simulink model "CIGRE_Islanded_1SM_2GFM_1GFL"  (R2020b)
settings: Solver=FixedStepAuto  StartTime=0.0  StopTime=simlt.T_stop  RelTol=1e-3
undefined symbols (not defined in the file): simlt
libraries: G2ELib_V1 x55, powerlib x19, powerlib_meascontrol x13, eePowerMeasurement x13
(part 1 of 2)
settings Model: Creator=keladaf  LastModifiedBy=keladaf
settings DataIOCC: ReturnWorkspaceOutputs=off
settings DebuggingCC: UnconnectedInputMsg=none  UnconnectedOutputMsg=none  UnconnectedLineMsg=none

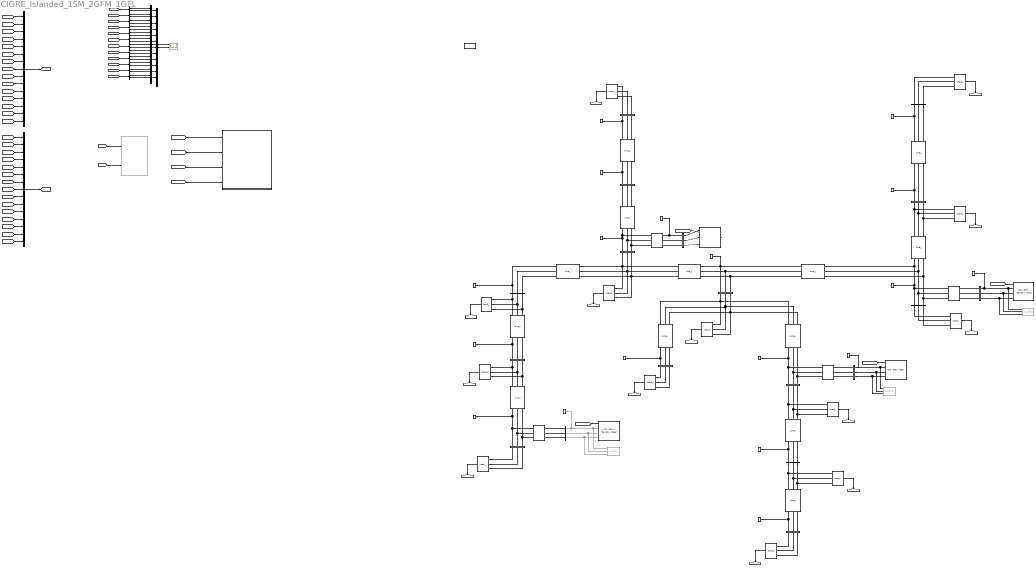
== system CIGRE_Islanded_1SM_2GFM_1GFL ==
  Bus Creator : BusCreator  Inputs=15
  Bus Creator1 : BusCreator  Inputs=15
  Bus Selector{,1..11} (12 alike) : BusSelector  OutputSignals=P_load,Q_load
  Bus_1 : G2ELib_V1/Miscellaneous Network Elements/Bus_i  VoltageMeasurement=phase-to-ground  SetLabelV=on  LabelV=V_Bus1  Vpu=off  VpuLL=off  CurrentMeasurement=yes  SetLabelI=on  LabelI=I_Bus1  Ipu=off  Pbase=100e6  Vbase=500e3  OutputType=Complex  PhasorSimulation=off  PSBequivalent=0
  Bus_10 : G2ELib_V1/Miscellaneous Network Elements/Bus_i  VoltageMeasurement=phase-to-ground  SetLabelV=on  LabelV=V_Bus10  Vpu=off  VpuLL=off  CurrentMeasurement=yes  SetLabelI=on  LabelI=I_Bus10  Ipu=off  Pbase=100e6  Vbase=500e3  OutputType=Complex  PhasorSimulation=off  PSBequivalent=0
  Bus_11 : G2ELib_V1/Miscellaneous Network Elements/Bus_i  VoltageMeasurement=phase-to-ground  SetLabelV=on  LabelV=V_Bus11  Vpu=off  VpuLL=off  CurrentMeasurement=yes  SetLabelI=on  LabelI=I_Bus11  Ipu=off  Pbase=100e6  Vbase=500e3  OutputType=Complex  PhasorSimulation=off  PSBequivalent=0
  Bus_12 : G2ELib_V1/Miscellaneous Network Elements/Bus_i  VoltageMeasurement=phase-to-ground  SetLabelV=on  LabelV=V_Bus12  Vpu=off  VpuLL=off  CurrentMeasurement=yes  SetLabelI=on  LabelI=I_Bus12  Ipu=off  Pbase=100e6  Vbase=500e3  OutputType=Complex  PhasorSimulation=off  PSBequivalent=0
  Bus_13 : G2ELib_V1/Miscellaneous Network Elements/Bus_i  VoltageMeasurement=phase-to-ground  SetLabelV=on  LabelV=V_Bus13  Vpu=off  VpuLL=off  CurrentMeasurement=yes  SetLabelI=on  LabelI=I_Bus13  Ipu=off  Pbase=100e6  Vbase=500e3  OutputType=Complex  PhasorSimulation=off  PSBequivalent=0
  Bus_14 : G2ELib_V1/Miscellaneous Network Elements/Bus_i  VoltageMeasurement=phase-to-ground  SetLabelV=on  LabelV=V_Bus14  Vpu=off  VpuLL=off  CurrentMeasurement=yes  SetLabelI=on  LabelI=I_Bus14  Ipu=off  Pbase=100e6  Vbase=500e3  OutputType=Complex  PhasorSimulation=off  PSBequivalent=0
  Bus_15 : G2ELib_V1/Miscellaneous Network Elements/Bus_i  VoltageMeasurement=phase-to-ground  SetLabelV=on  LabelV=V_Bus15  Vpu=off  VpuLL=off  CurrentMeasurement=yes  SetLabelI=on  LabelI=I_Bus15  Ipu=off  Pbase=100e6  Vbase=500e3  OutputType=Complex  PhasorSimulation=off  PSBequivalent=0
  Bus_16 : G2ELib_V1/Miscellaneous Network Elements/Bus_i  VoltageMeasurement=phase-to-ground  SetLabelV=on  LabelV=V_Bus16  Vpu=off  VpuLL=off  CurrentMeasurement=yes  SetLabelI=on  LabelI=I_Bus16  Ipu=off  Pbase=100e6  Vbase=500e3  OutputType=Complex  PhasorSimulation=off  PSBequivalent=0
  Bus_17 : G2ELib_V1/Miscellaneous Network Elements/Bus_i  VoltageMeasurement=phase-to-ground  SetLabelV=on  LabelV=V_Bus17  Vpu=off  VpuLL=off  CurrentMeasurement=yes  SetLabelI=on  LabelI=I_Bus17  Ipu=off  Pbase=100e6  Vbase=500e3  OutputType=Complex  PhasorSimulation=off  PSBequivalent=0
  Bus_18 : G2ELib_V1/Miscellaneous Network Elements/Bus_i  VoltageMeasurement=phase-to-ground  SetLabelV=on  LabelV=V_Bus18  Vpu=off  VpuLL=off  CurrentMeasurement=yes  SetLabelI=on  LabelI=I_Bus18  Ipu=off  Pbase=100e6  Vbase=500e3  OutputType=Complex  PhasorSimulation=off  PSBequivalent=0
  Bus_2 : G2ELib_V1/Miscellaneous Network Elements/Bus_i  VoltageMeasurement=phase-to-ground  SetLabelV=on  LabelV=V_Bus2  Vpu=off  VpuLL=off  CurrentMeasurement=yes  SetLabelI=on  LabelI=I_Bus2  Ipu=off  Pbase=100e6  Vbase=500e3  OutputType=Complex  PhasorSimulation=off  PSBequivalent=0
  Bus_3 : G2ELib_V1/Miscellaneous Network Elements/Bus_i  VoltageMeasurement=phase-to-ground  SetLabelV=on  LabelV=V_Bus3  Vpu=off  VpuLL=off  CurrentMeasurement=yes  SetLabelI=on  LabelI=I_Bus3  Ipu=off  Pbase=100e6  Vbase=500e3  OutputType=Complex  PhasorSimulation=off  PSBequivalent=0
  Bus_4 : G2ELib_V1/Miscellaneous Network Elements/Bus_i  VoltageMeasurement=phase-to-ground  SetLabelV=on  LabelV=V_Bus4  Vpu=off  VpuLL=off  CurrentMeasurement=yes  SetLabelI=on  LabelI=I_Bus4  Ipu=off  Pbase=100e6  Vbase=500e3  OutputType=Complex  PhasorSimulation=off  PSBequivalent=0
  Bus_5 : G2ELib_V1/Miscellaneous Network Elements/Bus_i  VoltageMeasurement=phase-to-ground  SetLabelV=on  LabelV=V_Bus5  Vpu=off  VpuLL=off  CurrentMeasurement=yes  SetLabelI=on  LabelI=I_Bus5  Ipu=off  Pbase=100e6  Vbase=500e3  OutputType=Complex  PhasorSimulation=off  PSBequivalent=0
  Bus_6 : G2ELib_V1/Miscellaneous Network Elements/Bus_i  VoltageMeasurement=phase-to-ground  SetLabelV=on  LabelV=V_Bus6  Vpu=off  VpuLL=off  CurrentMeasurement=yes  SetLabelI=on  LabelI=I_Bus6  Ipu=off  Pbase=100e6  Vbase=500e3  OutputType=Complex  PhasorSimulation=off  PSBequivalent=0
  Bus_7 : G2ELib_V1/Miscellaneous Network Elements/Bus_i  VoltageMeasurement=phase-to-ground  SetLabelV=on  LabelV=V_Bus7  Vpu=off  VpuLL=off  CurrentMeasurement=yes  SetLabelI=on  LabelI=I_Bus7  Ipu=off  Pbase=100e6  Vbase=500e3  OutputType=Complex  PhasorSimulation=off  PSBequivalent=0
  Bus_8 : G2ELib_V1/Miscellaneous Network Elements/Bus_i  VoltageMeasurement=phase-to-ground  SetLabelV=on  LabelV=V_Bus8  Vpu=off  VpuLL=off  CurrentMeasurement=yes  SetLabelI=on  LabelI=I_Bus8  Ipu=off  Pbase=100e6  Vbase=500e3  OutputType=Complex  PhasorSimulation=off  PSBequivalent=0
  Bus_9 : G2ELib_V1/Miscellaneous Network Elements/Bus_i  VoltageMeasurement=phase-to-ground  SetLabelV=on  LabelV=V_Bus9  Vpu=off  VpuLL=off  CurrentMeasurement=yes  SetLabelI=on  LabelI=I_Bus9  Ipu=off  Pbase=100e6  Vbase=500e3  OutputType=Complex  PhasorSimulation=off  PSBequivalent=0
  GFL_1 : G2ELib_V1/DC//AC Converters/Voltage Source Converters (VSC)/Grid-Following VSC (GFL)/VSC - GFL - Ideal  index_c=1  Parameters_fb=50  Parameters_wb=314.1593  GFL_Un=10000  GFL_Un_dc=16329.9316  GFL_Sn=2500000  GFL_Ib=204.1241  GFL_Ub=8164.9658  GFL_Ub_dc=16329.9316  GFL_Ib_dc=153.0931  GFL_Pref=0.7  GFL_Qref=0  GFL_V=0.98868  GFL_Theta_Eg0=-0.0027438  GFL_Vdcref=16329.9316  Delta_Pref_GFL=0.1  Tsw_Pref_GFL=1  Delta_Qref_GFL=0.1  Tsw_Qref_GFL=200  GFL_DC_link_R=500000  GFL_DC_link_C=0.05  GFL_DC_link_Vdc_init=16329.9316  DC_link_Tdc=1e-3  GFL_R1_pu=0.015  GFL_R2_pu=0.0533  GFL_L1_pu=0.1  GFL_L2_pu=0.00061115  GFL_C_pu=0.11  GFL_R1=0.6  GFL_R2=2.132  GFL_L1=0.012732  GFL_L2=7.7814e-05  GFL_C=8.7535e-06  Controllers=PLL  GFL_Control_PLL=1  GFL_Control_VIM=0  GFL_Control_SU_theta=1  GFL_Control_SU_omega=1  GFL_vdc_Kp=-319.9998  GFL_vdc_Ki=-9602.9001  GFL_KQ=-30  GFL_Inner_current_loop_Kp=0.17599  GFL_Inner_current_loop_Ki=57.3131  GFL_Inner_current_loop_Kffv=1  PLL_Kp=0.38197  PLL_Ki=22.9252  M_pll_0=-0.04362  VIM_wc=15.708  VIM_wc_ini=0  VIM_Iqd_sat=0.25  VIM_Rr_pu=0.0005  VIM_Lr_pu=0.05  VIM_Lm_pu=0.6  VIM_Rr=0.02  VIM_Lr=0.0063662  VIM_Lm=0.076394  VIM_Kp=3.1416  VIM_Kd=0.001  VIM_Nd=100  VIM_H=5.04  VIM_J=0.00025533  VIM_D=0.8  VIM_Inertia_ini=0  VIM_Ke_ini=0  VIM_T_sync=0  VIM_f0=50  VIM_w0=1  GFL_Inner_current_loop_Int_ini_d=0.01062  GFL_Inner_current_loop_Int_ini_q=0.0016313  GFL_Filter_I_ini="[ 21.80285     -136.1143      114.3114 ]"  GFL_Filter_V_ini="[ -22.149109     -6979.9183      7002.0674 ]"  GFL_Line_I_ini="[ -0.3965366     -124.9618      125.3584 ]"  GFL_Is0_dq0="[ 0.70802     0.10875           0 ]"  GFL_Eg0_dq0="[ 0.98868           0           0 ]"  GFL_Ig0_dq0="[ 0.70802           0           0 ]"  GFL_Vm0_dq0="[ 0.98842    0.072433           0 ]"  M_d_0=-7.3729e-05  M_q_0=-0.0036252  GFL_theta=-0.0027438
  GFM_1 : G2ELib_V1/DC//AC Converters/Voltage Source Converters (VSC)/Grid-Forming VSC (GFM)/VSC - GFM - Generic - Ideal  index_c=1  Parameters_fb=50  Parameters_wb=314.1593  GFM_Un=10000  GFM_Un_dc=16329.9316  GFM_Sn=2500000  GFM_Ib=204.1241  GFM_Ub=8164.9658  GFM_Ub_dc=16329.9316  GFM_Ib_dc=153.0931  GFM_Pref=0.7  GFM_Qref=0.40224  GFM_Vref=1  GFM_Theta_Eg0=-0.0039351  GFM_Vdcref=16329.9316  Delta_Pref_GFM=-0.1  Tsw_Pref_GFM=2  Delta_Vref_GFM=-0.01  Tsw_Vref_GFM=300  DC_link_R=500000  DC_link_C=0.05  DC_link_Vdc_init=16329.9316  DC_link_Tdc=1e-3  GFM_R1_pu=0.01  GFM_R2_pu=0.0533  GFM_L1_pu=0.1  GFM_L2_pu=0.00061115  GFM_C_pu=0.1  GFM_R1=0.4  GFM_R2=2.132  GFM_L1=0.012732  GFM_L2=7.7814e-05  GFM_C=7.9577e-06  Controllers=Droop  Control_PLL=0  Control_VIM=0  Control_MMU_QVDroop=1  Control_MMU_VSM=0  Control_dVOC=0  Control_MMU=1  Control_SU_PfDroop=1  Control_SU_Matching=0  Control_SU_VSM=0  Control_SU_theta=2  Control_SU_omega=2  Control_omega_set=2  Droop_mp=0.035  Droop_nq=0.0001  Droop_wc=2.5762  Droop_Int_ini=0  q_filter_wf=31.4159  q_filter_Int_ini=0.40224  p_filter_Int_ini=0.7  dVOC_eta=0.035  dVOC_alpha=5000  Matching_K_theta=112  VSM_D=28.5714  VSM_J=0.90946  VSM_AVR_Kp=0.05  VSM_AVR_Ki=11.64  VSM_Dq=10000  VSM_K=318.3099  Vdc_loop_Ki=0  Vdc_loop_Kp=3199.9998  Vdc_loop_Kffi=1  Vdc_loop_Int_ini=16329.9316  Damping_resistor_Enable=0  Damping_resistor_Rv=-0.052947  Damping_resistor_W_RV=62.8319  VI_Enable=0  VI_Rv_pu=0.01  VI_Lv_pu=0.1  TVI_K_RV=0.60041  TVI_Rho_XR=5  TVI_I_thresh_pu=1.2  Inner_voltage_loop_Kp=0.12732  Inner_voltage_loop_Ki=25.4725  Inner_voltage_loop_Kffi=1  Inner_current_loop_Kp=19.0886  Inner_current_loop_Ki=573130.8807  Inner_current_loop_Kffv=1  PLL_Kp=0.4  PLL_Ki=4.69  PLL_Int_ini=0  VIM_wc=0.1*2*pi*50  VIM_wc_ini=0  VIM_Iqd_sat=0.25  VIM_Rr_pu=0.0005  VIM_Lr_pu=0.05  VIM_Lm_pu=0.6  VIM_Rr=0.0048  VIM_Lr=0.0015  VIM_Lm=0.0183  VIM_Kp=3.1416  VIM_Kd=0.001  VIM_Nd=100  VIM_H=0  VIM_J=0.0043  VIM_D=10  VIM_Inertia_ini=0  VIM_Ke_ini=0  VIM_T_sync=0.01  VIM_f0=50.08  VIM_w0=1.0016  SFR_Enable=0  SFR_Rc=0.001  SFR_dP_max=0.3  Inner_voltage_loop_Int_ini_d=0  Inner_voltage_loop_Int_ini_q=-1.3878e-17  Inner_current_loop_Int_ini_d=0.007  Inner_current_loop_Int_ini_q=-0.0030224  Damping_resistor_Int_ini=0  Filter_I_ini="[ -62.25724     -92.40386      154.6611 ]"  Filter_V_ini="[ -32.129855     -7054.9481       7087.078 ]"  Line_I_ini="[ -82.6695     -82.12817      164.7977 ]"  Is0_dq0="[ 0.7    -0.30224           0 ]"  Eg0_dq0="[ 1           0           0 ]"  Ig0_dq0="[ 0.7    -0.40224           0 ]"  Vm0_dq0="[ 1.0372    0.066978           0 ]"  dVOC_ini_theta=-0.0039351  dVOC_ini_R0=[1,0;0,1]  Matching_Int_ini=-0.0039351  GFM_theta=-0.0039351
  GFM_2 : G2ELib_V1/DC//AC Converters/Voltage Source Converters (VSC)/Grid-Forming VSC (GFM)/VSC - GFM - Generic - Ideal  index_c=2  Parameters_fb=50  Parameters_wb=314.1593  GFM_Un=10000  GFM_Un_dc=16329.9316  GFM_Sn=2500000  GFM_Ib=204.1241  GFM_Ub=8164.9658  GFM_Ub_dc=16329.9316  GFM_Ib_dc=153.0931  GFM_Pref=0.7  GFM_Qref=0.20978  GFM_Vref=1  GFM_Theta_Eg0=0.0013498  GFM_Vdcref=16329.9316  Delta_Pref_GFM=-0.1  Tsw_Pref_GFM=2  Delta_Vref_GFM=-0.01  Tsw_Vref_GFM=300  DC_link_R=500000  DC_link_C=0.05  DC_link_Vdc_init=16329.9316  DC_link_Tdc=1e-3  GFM_R1_pu=0.01  GFM_R2_pu=0.0533  GFM_L1_pu=0.1  GFM_L2_pu=0.00061115  GFM_C_pu=0.1  GFM_R1=0.4  GFM_R2=2.132  GFM_L1=0.012732  GFM_L2=7.7814e-05  GFM_C=7.9577e-06  Controllers=Droop  Control_PLL=0  Control_VIM=0  Control_MMU_QVDroop=1  Control_MMU_VSM=0  Control_dVOC=0  Control_MMU=1  Control_SU_PfDroop=1  Control_SU_Matching=0  Control_SU_VSM=0  Control_SU_theta=2  Control_SU_omega=2  Control_omega_set=2  Droop_mp=0.035  Droop_nq=0.0001  Droop_wc=2.5762  Droop_Int_ini=0  q_filter_wf=31.4159  q_filter_Int_ini=0.20978  p_filter_Int_ini=0.7  dVOC_eta=0.035  dVOC_alpha=5000  Matching_K_theta=112  VSM_D=28.5714  VSM_J=0.90946  VSM_AVR_Kp=0.05  VSM_AVR_Ki=11.64  VSM_Dq=10000  VSM_K=318.3099  Vdc_loop_Ki=0  Vdc_loop_Kp=3199.9998  Vdc_loop_Kffi=1  Vdc_loop_Int_ini=16329.9316  Damping_resistor_Enable=0  Damping_resistor_Rv=-0.052947  Damping_resistor_W_RV=62.8319  VI_Enable=0  VI_Rv_pu=0.01  VI_Lv_pu=0.1  TVI_K_RV=0.60041  TVI_Rho_XR=5  TVI_I_thresh_pu=1.2  Inner_voltage_loop_Kp=0.12732  Inner_voltage_loop_Ki=25.4725  Inner_voltage_loop_Kffi=1  Inner_current_loop_Kp=19.0886  Inner_current_loop_Ki=573130.8807  Inner_current_loop_Kffv=1  PLL_Kp=0.4  PLL_Ki=4.69  PLL_Int_ini=0  VIM_wc=0.1*2*pi*50  VIM_wc_ini=0  VIM_Iqd_sat=0.25  VIM_Rr_pu=0.0005  VIM_Lr_pu=0.05  VIM_Lm_pu=0.6  VIM_Rr=0.0048  VIM_Lr=0.0015  VIM_Lm=0.0183  VIM_Kp=3.1416  VIM_Kd=0.001  VIM_Nd=100  VIM_H=0  VIM_J=0.0043  VIM_D=10  VIM_Inertia_ini=0  VIM_Ke_ini=0  VIM_T_sync=0.01  VIM_f0=50.08  VIM_w0=1.0016  SFR_Enable=0  SFR_Rc=0.001  SFR_dP_max=0.3  Inner_voltage_loop_Int_ini_d=0  Inner_voltage_loop_Int_ini_q=0  Inner_current_loop_Int_ini_d=0.007  Inner_current_loop_Int_ini_q=-0.0010978  Damping_resistor_Int_ini=0  Filter_I_ini="[ -22.21578     -112.6619      134.8777 ]"  Filter_V_ini="[ 11.021263      -7076.572      7065.5507 ]"  Line_I_ini="[ -42.62818     -102.4795      145.1077 ]"  Is0_dq0="[ 0.7    -0.10978           0 ]"  Eg0_dq0="[ 1  0  0 ]"  Ig0_dq0="[ 0.7    -0.20978           0 ]"  Vm0_dq0="[ 1.018    0.068902           0 ]"  dVOC_ini_theta=0.0013498  dVOC_ini_R0=[1,0;0,1]  Matching_Int_ini=0.0013498  GFM_theta=0.0013498
  Init_GFL_1 : G2ELib_V1/DC//AC Converters/Voltage Source Converters (VSC)/Grid-Following VSC (GFL)/Init_GFL_i  Commented=on  InternalConnection=Yg  VoltagePhases=off  Voltage=(10000)*0.988601  PhaseAngle=-0.17273  Voltage_phases=[25e3 25e3 25e3]/sqrt(3)  PhaseAngles_phases=[0 -120 +120]  Frequency=50  NonIdealSource=off  SpecifyImpedance=off  Resistance=0.8929  Inductance=16.58e-3  ShortCircuitLevel=100e6  BaseVoltage=10000  XRratio=7  BusType=PQ  Pref=1750000  Qref=0  Prefabc=[10e3, 10e3, 10e3]  Qrefabc=[0, 0, 0]  Qmin=-inf  Qmax=inf
  Init_GFM_1 : G2ELib_V1/DC//AC Converters/Voltage Source Converters (VSC)/Grid-Forming VSC (GFM)/Init_GFM_i  Commented=on  InternalConnection=Yg  VoltagePhases=off  Voltage=(10000)*1  PhaseAngle=-0.24228  Voltage_phases=[25e3 25e3 25e3]/sqrt(3)  PhaseAngles_phases=[0 -120 +120]  Frequency=50  NonIdealSource=off  SpecifyImpedance=off  Resistance=0.8929  Inductance=16.58e-3  ShortCircuitLevel=100e6  BaseVoltage=10000  XRratio=7  BusType=PV  Pref=1750000  Qref=1005611.7894  Prefabc=[10e3, 10e3, 10e3]  Qrefabc=[0, 0, 0]  Qmin=-inf  Qmax=inf
  Init_GFM_2 : G2ELib_V1/DC//AC Converters/Voltage Source Converters (VSC)/Grid-Forming VSC (GFM)/Init_GFM_i  Commented=on  InternalConnection=Yg  VoltagePhases=off  Voltage=(10000)*1  PhaseAngle=0.061558  Voltage_phases=[25e3 25e3 25e3]/sqrt(3)  PhaseAngles_phases=[0 -120 +120]  Frequency=50  NonIdealSource=off  SpecifyImpedance=off  Resistance=0.8929  Inductance=16.58e-3  ShortCircuitLevel=100e6  BaseVoltage=10000  XRratio=7  BusType=PV  Pref=1750000  Qref=524449.1246  Prefabc=[10e3, 10e3, 10e3]  Qrefabc=[0, 0, 0]  Qmin=-inf  Qmax=inf
  Line_1 : G2ELib_V1/Miscellaneous Network Elements/Line_i  LConnTagsString=a|b|c  RConnTagsString=A|B|C  Length=2.82  Frequency=50  Resistances=[ 0.501 0.3864 ]  Inductances=[ 0.0022791 0.0041264 ]  Capacitances=[ 1.5117e-07 7.751e-09 ]
      settings: AttributesFormatString=\n
  Line_10 : G2ELib_V1/Miscellaneous Network Elements/Line_i  LConnTagsString=a|b|c  RConnTagsString=A|B|C  Length=0.32  Frequency=50  Resistances=[ 0.501 0.3864 ]  Inductances=[ 0.0022791 0.0041264 ]  Capacitances=[ 1.5117e-07 7.751e-09 ]
      settings: AttributesFormatString=\n
  Line_11 : G2ELib_V1/Miscellaneous Network Elements/Line_i  LConnTagsString=a|b|c  RConnTagsString=A|B|C  Length=4.89  Frequency=50  Resistances=[ 0.51 0.3864 ]  Inductances=[ 0.001165 0.0041264 ]  Capacitances=[ 1.0097e-08 7.751e-09 ]
      settings: AttributesFormatString=\n
  Line_12 : G2ELib_V1/Miscellaneous Network Elements/Line_i  LConnTagsString=a|b|c  RConnTagsString=A|B|C  Length=2.99  Frequency=50  Resistances=[ 0.51 0.3864 ]  Inductances=[ 0.001165 0.0041264 ]  Capacitances=[ 1.0097e-08 7.751e-09 ]
      settings: AttributesFormatString=\n
  Line_13 : G2ELib_V1/Miscellaneous Network Elements/Line_i  LConnTagsString=a|b|c  RConnTagsString=A|B|C  Length=2  Frequency=50  Resistances=[ 0.51 0.3864 ]  Inductances=[ 0.001165 0.0041264 ]  Capacitances=[ 1.0097e-08 7.751e-09 ]
      settings: AttributesFormatString=\n
  Line_2 : G2ELib_V1/Miscellaneous Network Elements/Line_i  LConnTagsString=a|b|c  RConnTagsString=A|B|C  Length=4.42  Frequency=50  Resistances=[ 0.501 0.3864 ]  Inductances=[ 0.0022791 0.0041264 ]  Capacitances=[ 1.5117e-07 7.751e-09 ]
      settings: AttributesFormatString=\n
  Line_3 : G2ELib_V1/Miscellaneous Network Elements/Line_i  LConnTagsString=a|b|c  RConnTagsString=A|B|C  Length=0.61  Frequency=50  Resistances=[ 0.501 0.3864 ]  Inductances=[ 0.0022791 0.0041264 ]  Capacitances=[ 1.5117e-07 7.751e-09 ]
      settings: AttributesFormatString=\n
  Line_4 : G2ELib_V1/Miscellaneous Network Elements/Line_i  LConnTagsString=a|b|c  RConnTagsString=A|B|C  Length=0.56  Frequency=50  Resistances=[ 0.501 0.3864 ]  Inductances=[ 0.0022791 0.0041264 ]  Capacitances=[ 1.5117e-07 7.751e-09 ]
      settings: AttributesFormatString=\n
  Line_5 : G2ELib_V1/Miscellaneous Network Elements/Line_i  LConnTagsString=a|b|c  RConnTagsString=A|B|C  Length=1.54  Frequency=50  Resistances=[ 0.501 0.3864 ]  Inductances=[ 0.0022791 0.0041264 ]  Capacitances=[ 1.5117e-07 7.751e-09 ]
      settings: AttributesFormatString=\n
  Line_6 : G2ELib_V1/Miscellaneous Network Elements/Line_i  LConnTagsString=a|b|c  RConnTagsString=A|B|C  Length=1.3  Frequency=50  Resistances=[ 0.501 0.3864 ]  Inductances=[ 0.0022791 0.0041264 ]  Capacitances=[ 1.5117e-07 7.751e-09 ]
      settings: AttributesFormatString=\n
  Line_7 : G2ELib_V1/Miscellaneous Network Elements/Line_i  LConnTagsString=a|b|c  RConnTagsString=A|B|C  Length=1.67  Frequency=50  Resistances=[ 0.501 0.3864 ]  Inductances=[ 0.0022791 0.0041264 ]  Capacitances=[ 1.5117e-07 7.751e-09 ]
      settings: AttributesFormatString=\n
  Line_8 : G2ELib_V1/Miscellaneous Network Elements/Line_i  LConnTagsString=a|b|c  RConnTagsString=A|B|C  Length=0.24  Frequency=50  Resistances=[ 0.501 0.3864 ]  Inductances=[ 0.0022791 0.0041264 ]  Capacitances=[ 1.5117e-07 7.751e-09 ]
      settings: AttributesFormatString=\n
  Line_9 : G2ELib_V1/Miscellaneous Network Elements/Line_i  LConnTagsString=a|b|c  RConnTagsString=A|B|C  Length=0.77  Frequency=50  Resistances=[ 0.501 0.3864 ]  Inductances=[ 0.0022791 0.0041264 ]  Capacitances=[ 1.5117e-07 7.751e-09 ]
      settings: AttributesFormatString=\n
  Load Flow Bus1 : powerlib/Measurements/Load Flow Bus  LConnTagsString=a  Phases=single  Connectors=on one side  ID=BUS_1  Vbase=20000  Vref=1  Vangle=0  VLF=0.9759  VLFb=1  VLFc=1  angleLF=-1.897  angleLFb=0  angleLFc=0
  Load Flow Bus10 : powerlib/Measurements/Load Flow Bus  LConnTagsString=a  Phases=single  Connectors=on one side  ID=BUS_10  Vbase=20000  Vref=1  Vangle=0  VLF=0.9869  VLFb=1  VLFc=1  angleLF=-1.245  angleLFb=0  angleLFc=0
  Load Flow Bus11 : powerlib/Measurements/Load Flow Bus  LConnTagsString=a  Phases=single  Connectors=on one side  ID=BUS_11  Vbase=20000  Vref=1  Vangle=0  VLF=0.9865  VLFb=1  VLFc=1  angleLF=-1.266  angleLFb=0  angleLFc=0
  Load Flow Bus12 : powerlib/Measurements/Load Flow Bus  LConnTagsString=a  Phases=single  Connectors=on one side  ID=BUS_12  Vbase=20000  Vref=1  Vangle=0  VLF=0.9903  VLFb=1  VLFc=1  angleLF=-1.208  angleLFb=0  angleLFc=0
  Load Flow Bus13 : powerlib/Measurements/Load Flow Bus  LConnTagsString=a  Phases=single  Connectors=on one side  ID=BUS_13  Vbase=20000  Vref=1  Vangle=0  VLF=0.9839  VLFb=1  VLFc=1  angleLF=-1.348  angleLFb=0  angleLFc=0
  Load Flow Bus14 : powerlib/Measurements/Load Flow Bus  LConnTagsString=a  Phases=single  Connectors=on one side  ID=BUS_14  Vbase=20000  Vref=1  Vangle=0  VLF=0.9802  VLFb=1  VLFc=1  angleLF=-1.432  angleLFb=0  angleLFc=0
  Load Flow Bus15 : powerlib/Measurements/Load Flow Bus  LConnTagsString=a  Phases=single  Connectors=on one side  ID=BUS_15  Vbase=10000  Vref=1  Vangle=0  VLF=1  VLFb=1  VLFc=1  angleLF=0  angleLFb=0  angleLFc=0
  Load Flow Bus16 : powerlib/Measurements/Load Flow Bus  LConnTagsString=a  Phases=single  Connectors=on one side  ID=BUS_16  Vbase=10000  Vref=1  Vangle=0  VLF=1  VLFb=1  VLFc=1  angleLF=-0.2423  angleLFb=0  angleLFc=0
  Load Flow Bus17 : powerlib/Measurements/Load Flow Bus  LConnTagsString=a  Phases=single  Connectors=on one side  ID=BUS_17  Vbase=10000  Vref=1  Vangle=0  VLF=1  VLFb=1  VLFc=1  angleLF=0.06156  angleLFb=0  angleLFc=0
  Load Flow Bus18 : powerlib/Measurements/Load Flow Bus  LConnTagsString=a  Phases=single  Connectors=on one side  ID=BUS_18  Vbase=10000  Vref=1  Vangle=0  VLF=0.9886  VLFb=1  VLFc=1  angleLF=-0.1727  angleLFb=0  angleLFc=0
  Load Flow Bus2 : powerlib/Measurements/Load Flow Bus  LConnTagsString=a  Phases=single  Connectors=on one side  ID=BUS_2  Vbase=20000  Vref=1  Vangle=0  VLF=0.9819  VLFb=1  VLFc=1  angleLF=-1.603  angleLFb=0  angleLFc=0
  Load Flow Bus3 : powerlib/Measurements/Load Flow Bus  LConnTagsString=a  Phases=single  Connectors=on one side  ID=BUS_3  Vbase=20000  Vref=1  Vangle=0  VLF=0.9909  VLFb=1  VLFc=1  angleLF=-1.128  angleLFb=0  angleLFc=0
  Load Flow Bus4 : powerlib/Measurements/Load Flow Bus  LConnTagsString=a  Phases=single  Connectors=on one side  ID=BUS_4  Vbase=20000  Vref=1  Vangle=0  VLF=0.9913  VLFb=1  VLFc=1  angleLF=-1.106  angleLFb=0  angleLFc=0
  Load Flow Bus5 : powerlib/Measurements/Load Flow Bus  LConnTagsString=a  Phases=single  Connectors=on one side  ID=BUS_5  Vbase=20000  Vref=1  Vangle=0  VLF=0.992  VLFb=1  VLFc=1  angleLF=-1.064  angleLFb=0  angleLFc=0
  Load Flow Bus6 : powerlib/Measurements/Load Flow Bus  LConnTagsString=a  Phases=single  Connectors=on one side  ID=BUS_6  Vbase=20000  Vref=1  Vangle=0  VLF=0.9949  VLFb=1  VLFc=1  angleLF=-0.9022  angleLFb=0  angleLFc=0
  Load Flow Bus7 : powerlib/Measurements/Load Flow Bus  LConnTagsString=a  Phases=single  Connectors=on one side  ID=BUS_7  Vbase=20000  Vref=1  Vangle=0  VLF=0.986  VLFb=1  VLFc=1  angleLF=-1.241  angleLFb=0  angleLFc=0
  Load Flow Bus8 : powerlib/Measurements/Load Flow Bus  LConnTagsString=a  Phases=single  Connectors=on one side  ID=BUS_8  Vbase=20000  Vref=1  Vangle=0  VLF=0.9887  VLFb=1  VLFc=1  angleLF=-1.172  angleLFb=0  angleLFc=0
  Load Flow Bus9 : powerlib/Measurements/Load Flow Bus  LConnTagsString=a  Phases=single  Connectors=on one side  ID=BUS_9  Vbase=20000  Vref=1  Vangle=0  VLF=0.9886  VLFb=1  VLFc=1  angleLF=-1.156  angleLFb=0  angleLFc=0
  Load_1 : G2ELib_V1/Load Models/Load_i  SystemSampleTime=-1  VariantActivationTime=update diagram  Latency=0  AutoFrameSizeCalculation=off
      link override Dynamic Load: NominalVoltage=[ 20000 50 ]  ActiveReactivePowers=[0 0]  PositiveSequence=[0.975881 -1.89662]
      link override Series RLC Load: NominalVoltage=(20000)*0.975881  NominalFrequency=50  ActivePower=1200000  InductivePower=350000
      link override Step_P: StepV=15750000  StepT=250
      link override Step_Q: StepV=1150000  StepT=500
  Load_10 : G2ELib_V1/Load Models/Load_i  SystemSampleTime=-1  VariantActivationTime=update diagram  Latency=0  AutoFrameSizeCalculation=off
      link override Dynamic Load: NominalVoltage=[ 20000 50 ]  ActiveReactivePowers=[0 0]  PositiveSequence=[0.986487 -1.2658]
      link override Series RLC Load: NominalVoltage=(20000)*0.986487  NominalFrequency=50  ActivePower=750000  InductivePower=187970
      link override Step_P: StepV=15750000  StepT=250
      link override Step_Q: StepV=1150000  StepT=500
  Load_11 : G2ELib_V1/Load Models/Load_i  SystemSampleTime=-1  VariantActivationTime=update diagram  Latency=0  AutoFrameSizeCalculation=off
      link override Dynamic Load: NominalVoltage=[ 20000 50 ]  ActiveReactivePowers=[0 0]  PositiveSequence=[0.990287 -1.20828]
      link override Series RLC Load: NominalVoltage=(20000)*0.990287  NominalFrequency=50  ActivePower=605000  InductivePower=293010
      link override Step_P: StepV=15750000  StepT=250
      link override Step_Q: StepV=1150000  StepT=500
  Load_12 : G2ELib_V1/Load Models/Load_i  SystemSampleTime=-1  VariantActivationTime=update diagram  Latency=0  AutoFrameSizeCalculation=off
      link override Dynamic Load: NominalVoltage=[ 20000 50 ]  ActiveReactivePowers=[0 0]  PositiveSequence=[0.983916 -1.34769]
      link override Series RLC Load: NominalVoltage=(20000)*0.983916  NominalFrequency=50  ActivePower=40000  InductivePower=24790
      link override Step_P: StepV=15750000  StepT=250
      link override Step_Q: StepV=1150000  StepT=500
  Load_13 : G2ELib_V1/Load Models/Load_i  SystemSampleTime=-1  VariantActivationTime=update diagram  Latency=0  AutoFrameSizeCalculation=off
      link override Dynamic Load: NominalVoltage=[ 20000 50 ]  ActiveReactivePowers=[0 0]  PositiveSequence=[0.980235 -1.43176]
      link override Series RLC Load: NominalVoltage=(20000)*0.980235  NominalFrequency=50  ActivePower=800000  InductivePower=205000
      link override Step_P: StepV=15750000  StepT=250
      link override Step_Q: StepV=1150000  StepT=500
  Load_2 : G2ELib_V1/Load Models/Load_i  SystemSampleTime=-1  VariantActivationTime=update diagram  Latency=0  AutoFrameSizeCalculation=off
      link override Dynamic Load: NominalVoltage=[ 20000 50 ]  ActiveReactivePowers=[0 0]  PositiveSequence=[0.990895 -1.12776]
      link override Series RLC Load: NominalVoltage=(20000)*0.990895  NominalFrequency=50  ActivePower=550000  InductivePower=266380
      link override Step_P: StepV=15750000  StepT=250
      link override Step_Q: StepV=1150000  StepT=500
  Load_3 : G2ELib_V1/Load Models/Load_i  SystemSampleTime=-1  VariantActivationTime=update diagram  Latency=0  AutoFrameSizeCalculation=off
      link override Dynamic Load: NominalVoltage=[ 20000 50 ]  ActiveReactivePowers=[0 0]  PositiveSequence=[0.99126 -1.10596]
      link override Series RLC Load: NominalVoltage=(20000)*0.99126  NominalFrequency=50  ActivePower=445000  InductivePower=111530
      link override Step_P: StepV=15750000  StepT=250
      link override Step_Q: StepV=1150000  StepT=500
  Load_4 : G2ELib_V1/Load Models/Load_i  SystemSampleTime=-1  VariantActivationTime=update diagram  Latency=0  AutoFrameSizeCalculation=off
      link override Dynamic Load: NominalVoltage=[ 20000 50 ]  ActiveReactivePowers=[0 0]  PositiveSequence=[0.992012 -1.06407]
      link override Series RLC Load: NominalVoltage=(20000)*0.992012  NominalFrequency=50  ActivePower=340000  InductivePower=85210
      link override Step_P: StepV=15750000  StepT=250
      link override Step_Q: StepV=1150000  StepT=500
  Load_5 : G2ELib_V1/Load Models/Load_i  SystemSampleTime=-1  VariantActivationTime=update diagram  Latency=0  AutoFrameSizeCalculation=off
      link override Dynamic Load: NominalVoltage=[ 20000 50 ]  ActiveReactivePowers=[0 0]  PositiveSequence=[0.994928 -0.902162]
      link override Series RLC Load: NominalVoltage=(20000)*0.994928  NominalFrequency=50  ActivePower=570000  InductivePower=276060
      link override Step_P: StepV=15750000  StepT=250
      link override Step_Q: StepV=1150000  StepT=500
  Load_6 : G2ELib_V1/Load Models/Load_i  SystemSampleTime=-1  VariantActivationTime=update diagram  Latency=0  AutoFrameSizeCalculation=off
      link override Dynamic Load: NominalVoltage=[ 20000 50 ]  ActiveReactivePowers=[0 0]  PositiveSequence=[0.986046 -1.24096]
      link override Series RLC Load: NominalVoltage=(20000)*0.986046  NominalFrequency=50  ActivePower=675000  InductivePower=418330
      link override Step_P: StepV=15750000  StepT=250
      link override Step_Q: StepV=1150000  StepT=500
  Load_7 : G2ELib_V1/Load Models/Load_i  SystemSampleTime=-1  VariantActivationTime=update diagram  Latency=0  AutoFrameSizeCalculation=off
      link override Dynamic Load: NominalVoltage=[ 20000 50 ]  ActiveReactivePowers=[0 0]  PositiveSequence=[0.988701 -1.17183]
      link override Series RLC Load: NominalVoltage=(20000)*0.988701  NominalFrequency=50  ActivePower=605000  InductivePower=151630
      link override Step_P: StepV=15750000  StepT=250
      link override Step_Q: StepV=1150000  StepT=500
  Load_8 : G2ELib_V1/Load Models/Load_i  SystemSampleTime=-1  VariantActivationTime=update diagram  Latency=0  AutoFrameSizeCalculation=off
      link override Dynamic Load: NominalVoltage=[ 20000 50 ]  ActiveReactivePowers=[0 0]  PositiveSequence=[0.988629 -1.1563]
      link override Series RLC Load: NominalVoltage=(20000)*0.988629  NominalFrequency=50  ActivePower=90000  InductivePower=55780
      link override Step_P: StepV=15750000  StepT=250
      link override Step_Q: StepV=1150000  StepT=500
  Load_9 : G2ELib_V1/Load Models/Load_i  SystemSampleTime=-1  VariantActivationTime=update diagram  Latency=0  AutoFrameSizeCalculation=off
      link override Dynamic Load: NominalVoltage=[ 20000 50 ]  ActiveReactivePowers=[0 0]  PositiveSequence=[0.986899 -1.24487]
      link override Series RLC Load: NominalVoltage=(20000)*0.986899  NominalFrequency=50  ActivePower=565000  InductivePower=141600
      link override Step_P: StepV=15750000  StepT=250
      link override Step_Q: StepV=1150000  StepT=500
  Loads scope : Scope  Commented=on  NumInputPorts=2
  Mux : Mux  Inputs=13
  Mux1 : Mux  Inputs=13
  Network scopes : Subsystem  Commented=on
  SM_1 : G2ELib_V1/Synchronous Machine Models/Simulink - Synchronous Machine - Full Controls  index_SM=1  SM_Sn=2500000  SM_Un=10000  Parameters_fb=50  SM_wr=1  SM_Ra=0.003  SM_Ll=0.15  SM_Lad=1.66  SM_Laq=1.61  SM_L1d=0.1713  SM_R1d=0.0284  SM_L1q=0.7252  SM_R1q=0.00619  SM_L2q=0.125  SM_R2q=0.02368  SM_Rfd=0.0006  SM_Lfd=0.165  SM_H=5  SM_K_D=0  SM_Es_base=8164.9658  SM_Is_base=204.1241  SM_Pt=0.80675  SM_Qt=0.37935  SM_Et=1  SM_It=0.89149  SM_Te_0=0.80913  SM_alpha=0  SM_Phi=0  SM_delta0=0.70421  SM_theta_0=-0.86659  SM_ed_0=0.64743  SM_eq_0=0.76212  SM_id_0=0.81143  SM_iq_0=0.36924  SM_efd_0=2.2319  SM_ifd_0=1.3445  SM_Psi_d0=0.76323  SM_Psi_q0=-0.64986  SM_Psi_fd0=1.1068  SM_Psi_1d0=0.88495  SM_Psi_1q0=-0.59448  SM_Psi_2q0=-0.59448  SM_mp=0.5  SM_Tg=0.2  SM_Tr=0.02  SM_Ka=300  SM_Ta=0.001  SM_Ke=1  SM_Te=0.0001  SM_Tb=0  SM_Tc=0  SM_Kf=0.001  SM_Tf=0.1  SM_Efmin=-11.5  SM_Efmax=11.5  SM_Kp=0  SM_T_LP=0.03  SM_K_PSS=2  SM_T_HP=2  SM_T1n=0.05  SM_T1d=0.02  SM_T2n=3  SM_T2d=5.4  SM_VSmax=0.15  SM_VSmin=-0.15  delta_Pref=0.1  T_Pref=200  delta_Vref=0.01  T_Vref=200
      link override Excitation System: v0=[1 2.2952]
      link override Synchronous Machine pu Fundamental: BusType=swing  InitialConditions=[0 -48.0116 0.937893 0.937893 0.937893 -24.0058 -144.006 95.9942 2.29518]
      link override Three-Phase Parallel RLC Load: NominalVoltage=(10000)*1
  Subsystem : Subsystem
  Transformer_{1..4} (4 alike) : G2ELib_V1/Miscellaneous Network Elements/Transformer_i  Winding1Connection=Yg  Winding2Connection=Yg  CoreType=Three single-phase transformers  SetSaturation=off  Hysteresis=off  DataFile='hysteresis'  SetInitialFlux=off  Measurements=None  UNITS=pu  NominalPower=[ 2500000 50 ]  Winding1=[ 20000 0.0001 0.012 ]  Winding2=[ 10000 0.0001 0.012 ]  Rm=500  Lm=500  L0=0.5  Saturation=[ 0,0 ; 0.0024,1.2 ; 1.0,1.52 ]  InitialFluxes=[ 0.8 , -0.8 , 0.7 ]  BreakLoop=off  DiscreteSolver=Trapezoidal iterative  DataType=off  TransfoNumber=1
  powergui : powerlib/powergui  Priority=1  SimulationMode=Discrete  SampleTime=simlt.T_step  frequency=60  Iterations=50  frequencyindice=50  Pbase=5e6  ErrMax=0.0001  UnitsV=kV  UnitsW=MW  buscounter=0  FunctionMessages=off  echomessages=off  EnableUseOfTLC=off  CurrentSourceSwitches=off  DisableSnubberDevices=off  DisableRonSwitches=off  DisableVfSwitches=off  DisplayEquations=off  AutomaticDiscreteSolvers=off  SolverType=Tustin/Backward Euler (TBE)  Interpol=off  ExternalGateDelay=off  methode=off  Ts=100  x0status=blocks  SPID=on  SwTol=0  HookPort=off  NonlinearTolerance=1e-4  nMaxIteration=100  ContinueOnMaxIteration=off  RestoreLinks=warning  ResistiveCurrentMeasurement=off  Frange=[0:2:500]  Ylog=off  Xlog=on  ShowGrid=off  save=off  variable=ZData  structure=Fluxes  ZoomFFT=off  StartTime=0.05  cycles=5  DisplayStyle=1  fundamental=50  FreqAxis=off  MaxFrequency=300  frequencyindicesteady=1  RmsSteady=1  display=off
  wires:
  Bus Creator/1 -> [V_buses]
  [V_Bus1] -> Bus Creator/1  "V1"
  [V_Bus2] -> Bus Creator/2  "V2"
  [V_Bus3] -> Bus Creator/3  "V3"
  [V_Bus4] -> Bus Creator/4  "V4"
  [V_Bus5] -> Bus Creator/5  "V5"
  [V_Bus6] -> Bus Creator/6  "V6"
  [V_Bus7] -> Bus Creator/7  "V7"
  [V_Bus8] -> Bus Creator/8  "V8"
  [V_Bus9] -> Bus Creator/9  "V9"
  [V_Bus10] -> Bus Creator/10  "V10"
  [V_Bus11] -> Bus Creator/11  "V11"
  [V_Bus12] -> Bus Creator/12  "V12"
  [V_Bus13] -> Bus Creator/13  "V13"
  [V_Bus14] -> Bus Creator/14  "V14"
  [V_Bus15] -> Bus Creator/15  "V15"
  [I_Bus15] -> Bus Creator1/15  "I15"
  [I_Bus14] -> Bus Creator1/14  "I14"
  [I_Bus13] -> Bus Creator1/13  "I13"
  [I_Bus12] -> Bus Creator1/12  "I12"
  [I_Bus11] -> Bus Creator1/11  "I11"
  [I_Bus10] -> Bus Creator1/10  "I10"
  [I_Bus9] -> Bus Creator1/9  "I9"
  [I_Bus8] -> Bus Creator1/8  "I8"
  [I_Bus7] -> Bus Creator1/7  "I7"
  [I_Bus6] -> Bus Creator1/6  "I6"
  [I_Bus5] -> Bus Creator1/5  "I5"
  [I_Bus4] -> Bus Creator1/4  "I4"
  [I_Bus3] -> Bus Creator1/3  "I3"
  [I_Bus2] -> Bus Creator1/2  "I2"
  [I_Bus1] -> Bus Creator1/1  "I1"
  Bus Creator1/1 -> [I_buses]
  [V_buses] -> Network scopes/1(V_buses)
  [I_buses] -> Network scopes/2(I_buses)
  [PQ_Load1] -> Bus Selector/1
  [PQ_Load3] -> Bus Selector1/1
  Bus Selector/1 -> Mux/1  "<P_load>"
  Bus Selector1/1 -> Mux/2  "<P_load>"
  Bus Selector2/1 -> Mux/3  "<P_load>"
  Bus Selector3/1 -> Mux/4  "<P_load>"
  Bus Selector4/1 -> Mux/5  "<P_load>"
  Bus Selector5/1 -> Mux/6  "<P_load>"
  Bus Selector6/1 -> Mux/7  "<P_load>"
  Bus Selector7/1 -> Mux/8  "<P_load>"
  Bus Selector8/1 -> Mux/9  "<P_load>"
  Bus Selector9/1 -> Mux/10  "<P_load>"
  Bus Selector10/1 -> Mux/11  "<P_load>"
  Bus Selector11/1 -> Mux/12  "<P_load>"
  Bus Selector/2 -> Mux1/1  "<Q_load>"
  Bus Selector1/2 -> Mux1/2  "<Q_load>"
  Bus Selector2/2 -> Mux1/3  "<Q_load>"
  Bus Selector3/2 -> Mux1/4  "<Q_load>"
  Bus Selector4/2 -> Mux1/5  "<Q_load>"
  Bus Selector5/2 -> Mux1/6  "<Q_load>"
  Bus Selector6/2 -> Mux1/7  "<Q_load>"
  Bus Selector7/2 -> Mux1/8  "<Q_load>"
  Bus Selector8/2 -> Mux1/9  "<Q_load>"
  Bus Selector9/2 -> Mux1/10  "<Q_load>"
  Bus Selector10/2 -> Mux1/11  "<Q_load>"
  Bus Selector11/2 -> Mux1/12  "<Q_load>"
  Mux/1 -> Loads scope/1
  Mux1/1 -> Loads scope/2
  [PQ_Load4] -> Bus Selector2/1
  [PQ_Load5] -> Bus Selector3/1
  [PQ_Load6] -> Bus Selector4/1
  [PQ_Load7] -> Bus Selector5/1
  [PQ_Load8] -> Bus Selector6/1
  [PQ_Load9] -> Bus Selector7/1
  [PQ_Load10] -> Bus Selector8/1
  [PQ_Load11] -> Bus Selector9/1
  [PQ_Load12] -> Bus Selector10/1
  [PQ_Load13] -> Bus Selector11/1
  Load_1/1 -> [PQ_Load1]
  Load_2/1 -> [PQ_Load2]
  Load_3/1 -> [PQ_Load3]
  Load_4/1 -> [PQ_Load4]
  Load_5/1 -> [PQ_Load5]
  Load_6/1 -> [PQ_Load6]
  Load_7/1 -> [PQ_Load7]
  Load_8/1 -> [PQ_Load8]
  Load_9/1 -> [PQ_Load9]
  Load_10/1 -> [PQ_Load10]
  Load_11/1 -> [PQ_Load11]
  Load_12/1 -> [PQ_Load12]
  Load_13/1 -> [PQ_Load13]
  SM_1/1 -> [SM1_measurements]
  GFM_1/1 -> [GFM1_measurements]
  GFM_2/1 -> [GFM2_measurements]
  GFL_1/1 -> [GFL1_measurements]
  [SM1_measurements] -> Subsystem/1(SM_1)
  [GFM1_measurements] -> Subsystem/2(GFM_1)
  [GFM2_measurements] -> Subsystem/3(GFM_2)
  [GFL1_measurements] -> Subsystem/4(GFL_1)
  connections:
  Line_1/RConn1 -- Load Flow Bus1/LConn1 -- Bus_1/LConn1
  Line_1/RConn2 -- Bus_1/LConn2
  Line_1/RConn3 -- Bus_1/LConn3
  Bus_2/RConn1 -- Load Flow Bus2/LConn1 -- Line_1/LConn1
  Bus_2/RConn2 -- Line_1/LConn2
  Bus_2/RConn3 -- Line_1/LConn3
  Line_2/RConn1 -- Bus_2/LConn1
  Line_2/RConn2 -- Bus_2/LConn2
  Line_2/RConn3 -- Bus_2/LConn3
  Load_1/LConn1 -- Bus_1/RConn1
  Load_1/LConn2 -- Bus_1/RConn2
  Load_1/LConn3 -- Bus_1/RConn3
  Bus_3/RConn1 -- Load Flow Bus3/LConn1 -- Line_2/LConn1 -- Transformer_1/LConn1
  Bus_3/RConn3 -- Line_2/LConn3 -- Transformer_1/LConn3
  Bus_3/RConn2 -- Line_2/LConn2 -- Transformer_1/LConn2
  Line_3/RConn1 -- Line_6/LConn1 -- Bus_3/LConn1 -- Load_2/LConn1
  Line_3/LConn1 -- Load Flow Bus4/LConn1 -- Bus_4/RConn1
  Line_3/LConn2 -- Bus_4/RConn2
  Line_3/RConn2 -- Line_6/LConn2 -- Bus_3/LConn2 -- Load_2/LConn2
  Line_3/RConn3 -- Line_6/LConn3 -- Bus_3/LConn3 -- Load_2/LConn3
  Line_3/LConn3 -- Bus_4/RConn3
  Line_4/RConn1 -- Load_3/LConn1 -- Bus_4/LConn1
  Line_4/RConn2 -- Load_3/LConn2 -- Bus_4/LConn2
  Line_4/RConn3 -- Bus_4/LConn3 -- Load_3/LConn3
  Bus_5/RConn1 -- Line_4/LConn1 -- Load Flow Bus5/LConn1
  Bus_5/RConn2 -- Line_4/LConn2
  Bus_5/RConn3 -- Line_4/LConn3
  Line_5/RConn1 -- Load_4/LConn1 -- Bus_5/LConn1
  Line_5/RConn2 -- Load_4/LConn2 -- Bus_5/LConn2
  Line_5/RConn3 -- Bus_5/LConn3 -- Load_4/LConn3
  Bus_6/RConn2 -- Line_5/LConn2 -- Transformer_3/LConn2
  Bus_6/RConn3 -- Transformer_3/LConn3 -- Line_5/LConn3
  Bus_6/RConn1 -- Load Flow Bus6/LConn1 -- Line_5/LConn1 -- Transformer_3/LConn1
  Load_5/LConn1 -- Bus_6/LConn1
  Load_5/LConn2 -- Bus_6/LConn2
  Load_5/LConn3 -- Bus_6/LConn3
  Load_6/LConn1 -- Bus_7/LConn1
  Load_6/LConn2 -- Bus_7/LConn2
  Load_6/LConn3 -- Bus_7/LConn3
  Line_6/RConn1 -- Load Flow Bus8/LConn1 -- Line_13/LConn1 -- Bus_8/RConn1
  Line_6/RConn2 -- Line_13/LConn2 -- Bus_8/RConn2
  Line_6/RConn3 -- Line_13/LConn3 -- Bus_8/RConn3
  Line_7/LConn1 -- Load Flow Bus7/LConn1 -- Bus_7/RConn1
  Line_7/LConn2 -- Bus_7/RConn2
  Line_7/LConn3 -- Bus_7/RConn3
  Line_7/RConn1 -- Line_8/RConn1 -- Bus_8/LConn1 -- Load_7/LConn1
  Line_7/RConn2 -- Line_8/RConn2 -- Bus_8/LConn2 -- Load_7/LConn2
  Line_7/RConn3 -- Load_7/LConn3 -- Line_8/RConn3 -- Bus_8/LConn3
  Bus_9/RConn2 -- Line_8/LConn2 -- Transformer_4/LConn2
  Bus_9/RConn1 -- Line_8/LConn1 -- Load Flow Bus9/LConn1 -- Transformer_4/LConn1
  Bus_9/RConn3 -- Line_8/LConn3 -- Transformer_4/LConn3
  Line_9/RConn1 -- Bus_9/LConn1 -- Load_8/LConn1
  Line_9/RConn2 -- Bus_9/LConn2 -- Load_8/LConn2
  Line_9/RConn3 -- Load_8/LConn3 -- Bus_9/LConn3
  Bus_10/RConn1 -- Load Flow Bus10/LConn1 -- Line_9/LConn1
  Bus_10/RConn2 -- Line_9/LConn2
  Bus_10/RConn3 -- Line_9/LConn3
  Bus_10/LConn1 -- Load_9/LConn1 -- Line_10/RConn1
  Line_10/RConn2 -- Load_9/LConn2 -- Bus_10/LConn2
  Bus_10/LConn3 -- Load_9/LConn3 -- Line_10/RConn3
  Bus_11/RConn2 -- Line_10/LConn2
  Bus_11/RConn3 -- Line_10/LConn3
  Bus_11/RConn1 -- Load Flow Bus11/LConn1 -- Line_10/LConn1
  Load_10/LConn1 -- Bus_11/LConn1
  Load_10/LConn2 -- Bus_11/LConn2
  Load_10/LConn3 -- Bus_11/LConn3
  Line_11/LConn1 -- Line_13/RConn1 -- Load Flow Bus12/LConn1 -- Transformer_2/LConn1 -- Bus_12/RConn1
  Line_11/LConn2 -- Line_13/RConn2 -- Transformer_2/LConn2 -- Bus_12/RConn2
  Line_11/LConn3 -- Bus_12/RConn3 -- Transformer_2/LConn3 -- Line_13/RConn3
  Bus_13/LConn2 -- Line_11/RConn2 -- Load_12/LConn2
  Bus_13/LConn1 -- Load_12/LConn1 -- Line_11/RConn1
  Bus_13/LConn3 -- Line_11/RConn3 -- Load_12/LConn3
  Line_12/LConn2 -- Bus_13/RConn2
  Line_12/LConn1 -- Load Flow Bus13/LConn1 -- Bus_13/RConn1
  Line_12/LConn3 -- Bus_13/RConn3
  Bus_14/LConn1 -- Load Flow Bus14/LConn1 -- Line_12/RConn1
  Bus_14/LConn2 -- Line_12/RConn2
  Bus_14/LConn3 -- Line_12/RConn3
  Load_11/LConn1 -- Bus_12/LConn1
  Load_11/LConn2 -- Bus_12/LConn2
  Load_11/LConn3 -- Bus_12/LConn3
  Load_13/LConn1 -- Bus_14/RConn1
  Load_13/LConn2 -- Bus_14/RConn2
  Load_13/LConn3 -- Bus_14/RConn3
  Bus_15/RConn1 -- SM_1/LConn1
  Bus_15/RConn2 -- SM_1/LConn2
  SM_1/LConn3 -- Bus_15/RConn3
  Bus_15/LConn1 -- Load Flow Bus15/LConn1 -- Transformer_1/RConn1
  Bus_15/LConn2 -- Transformer_1/RConn2
  Bus_15/LConn3 -- Transformer_1/RConn3
  Bus_16/LConn2 -- Transformer_2/RConn2
  Bus_16/LConn1 -- Transformer_2/RConn1
  GFM_1/RConn3 -- Init_GFM_1/RConn3 -- Bus_16/RConn3
  GFM_1/RConn1 -- Init_GFM_1/RConn1 -- Load Flow Bus16/LConn1 -- Bus_16/RConn1
  GFM_1/RConn2 -- Init_GFM_1/RConn2 -- Bus_16/RConn2
  Bus_16/LConn3 -- Transformer_2/RConn3
  Init_GFM_2/RConn3 -- GFM_2/RConn3 -- Bus_17/RConn3
  Init_GFM_2/RConn1 -- GFM_2/RConn1 -- Load Flow Bus17/LConn1 -- Bus_17/RConn1
  Init_GFM_2/RConn2 -- GFM_2/RConn2 -- Bus_17/RConn2
  Bus_17/LConn3 -- Transformer_3/RConn3
  Bus_17/LConn1 -- Transformer_3/RConn1
  Bus_17/LConn2 -- Transformer_3/RConn2
  GFL_1/RConn3 -- Bus_18/RConn3 -- Init_GFL_1/RConn3
  GFL_1/RConn2 -- Bus_18/RConn2 -- Init_GFL_1/RConn2
  GFL_1/RConn1 -- Load Flow Bus18/LConn1 -- Bus_18/RConn1 -- Init_GFL_1/RConn1
  Bus_18/LConn1 -- Transformer_4/RConn1
  Bus_18/LConn2 -- Transformer_4/RConn2
  Bus_18/LConn3 -- Transformer_4/RConn3

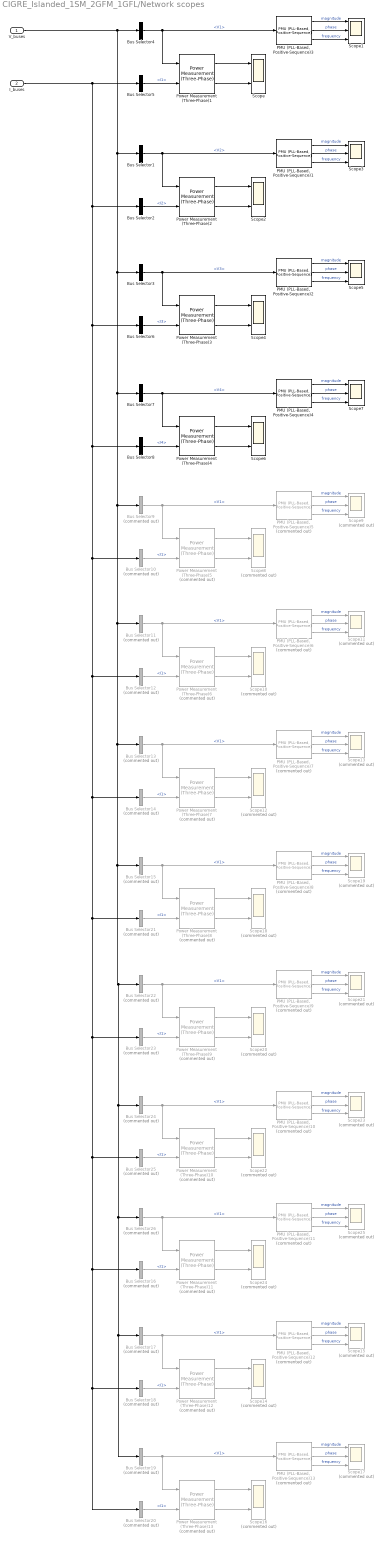
== system CIGRE_Islanded_1SM_2GFM_1GFL/Network scopes ==
  V_buses : Inport
  I_buses : Inport  Port=2
  Bus Selector1 : BusSelector  OutputSignals=V2
  Bus Selector{10,12,14,16,18,20..21,23,25} (9 alike) : BusSelector  Commented=on  OutputSignals=I1
  Bus Selector{9,11,13,15,17,19,22,24,26} (9 alike) : BusSelector  Commented=on  OutputSignals=V1
  Bus Selector2 : BusSelector  OutputSignals=I2
  Bus Selector3 : BusSelector  OutputSignals=V3
  Bus Selector4 : BusSelector  OutputSignals=V1
  Bus Selector5 : BusSelector  OutputSignals=I1
  Bus Selector6 : BusSelector  OutputSignals=I3
  Bus Selector7 : BusSelector  OutputSignals=V4
  Bus Selector8 : BusSelector  OutputSignals=I4
  PMU (PLL-Based, Positive-Sequence){1..4} (4 alike) : powerlib_meascontrol/Measurements/PMU (PLL-Based, Positive-Sequence)  nominalFrequency=50  samplingRate=64  reportingFactor=1
      settings: SourceProductBaseCode=PS
  PMU (PLL-Based, Positive-Sequence){5..13} (9 alike) : powerlib_meascontrol/Measurements/PMU (PLL-Based, Positive-Sequence)  Commented=on  nominalFrequency=50  samplingRate=64  reportingFactor=1
      settings: SourceProductBaseCode=PS
  Power Measurement (Three-Phase){1..4} (4 alike) : eePowerMeasurement/Power Measurement (Three-Phase)  LabelModeActiveChoice=Continuous  F=50  K=1  Seq=Positive  Ts=0
      settings: SourceProductBaseCode=PS
  Power Measurement (Three-Phase){5..13} (9 alike) : eePowerMeasurement/Power Measurement (Three-Phase)  Commented=on  LabelModeActiveChoice=Continuous  F=50  K=1  Seq=Positive  Ts=0
      settings: SourceProductBaseCode=PS
  Scope{,2,4,6} (4 alike) : Scope  NumInputPorts=2
  Scope{1,3,5,7} (4 alike) : Scope  NumInputPorts=3
  Scope{8,10,12,14,16,18,20,22,24} (9 alike) : Scope  Commented=on  NumInputPorts=2
  Scope{9,11,13,15,17,19,21,23,25} (9 alike) : Scope  Commented=on  NumInputPorts=3
  wires:
  I_buses/1 -> Bus Selector23/1, Bus Selector20/1, Bus Selector18/1, Bus Selector16/1, Bus Selector25/1, Bus Selector21/1, Bus Selector14/1, Bus Selector12/1, Bus Selector10/1, Bus Selector8/1, Bus Selector6/1, Bus Selector2/1, Bus Selector5/1
  V_buses/1 -> Bus Selector19/1, Bus Selector17/1, Bus Selector26/1, Bus Selector24/1, Bus Selector22/1, Bus Selector15/1, Bus Selector13/1, Bus Selector11/1, Bus Selector9/1, Bus Selector7/1, Bus Selector3/1, Bus Selector1/1, Bus Selector4/1
  Bus Selector5/1 -> Power Measurement (Three-Phase)1/2  "<I1>"
  "PMU (PLL-Based, Positive-Sequence)3"/2 -> Scope1/2  "phase"
  Bus Selector4/1 -> Power Measurement (Three-Phase)1/1, "PMU (PLL-Based, Positive-Sequence)3"/1  "<V1>"
  Power Measurement (Three-Phase)1/2 -> Scope/2
  "PMU (PLL-Based, Positive-Sequence)3"/3 -> Scope1/3  "frequency"
  "PMU (PLL-Based, Positive-Sequence)3"/1 -> Scope1/1  "magnitude"
  Power Measurement (Three-Phase)1/1 -> Scope/1
  Power Measurement (Three-Phase)2/1 -> Scope2/1
  "PMU (PLL-Based, Positive-Sequence)1"/1 -> Scope3/1  "magnitude"
  "PMU (PLL-Based, Positive-Sequence)1"/3 -> Scope3/3  "frequency"
  Power Measurement (Three-Phase)2/2 -> Scope2/2
  Bus Selector1/1 -> "PMU (PLL-Based, Positive-Sequence)1"/1, Power Measurement (Three-Phase)2/1  "<V2>"
  "PMU (PLL-Based, Positive-Sequence)1"/2 -> Scope3/2  "phase"
  Bus Selector2/1 -> Power Measurement (Three-Phase)2/2  "<I2>"
  Bus Selector6/1 -> Power Measurement (Three-Phase)3/2  "<I3>"
  "PMU (PLL-Based, Positive-Sequence)2"/2 -> Scope5/2  "phase"
  Bus Selector3/1 -> Power Measurement (Three-Phase)3/1, "PMU (PLL-Based, Positive-Sequence)2"/1  "<V3>"
  Power Measurement (Three-Phase)3/2 -> Scope4/2
  "PMU (PLL-Based, Positive-Sequence)2"/3 -> Scope5/3  "frequency"
  "PMU (PLL-Based, Positive-Sequence)2"/1 -> Scope5/1  "magnitude"
  Power Measurement (Three-Phase)3/1 -> Scope4/1
  Power Measurement (Three-Phase)4/1 -> Scope6/1
  "PMU (PLL-Based, Positive-Sequence)4"/1 -> Scope7/1  "magnitude"
  "PMU (PLL-Based, Positive-Sequence)4"/3 -> Scope7/3  "frequency"
  Power Measurement (Three-Phase)4/2 -> Scope6/2
  Bus Selector7/1 -> "PMU (PLL-Based, Positive-Sequence)4"/1, Power Measurement (Three-Phase)4/1  "<V4>"
  "PMU (PLL-Based, Positive-Sequence)4"/2 -> Scope7/2  "phase"
  Bus Selector8/1 -> Power Measurement (Three-Phase)4/2  "<I4>"
  Bus Selector14/1 -> Power Measurement (Three-Phase)7/2  "<I1>"
  "PMU (PLL-Based, Positive-Sequence)7"/2 -> Scope13/2  "phase"
  Bus Selector13/1 -> Power Measurement (Three-Phase)7/1, "PMU (PLL-Based, Positive-Sequence)7"/1  "<V1>"
  Power Measurement (Three-Phase)7/2 -> Scope12/2
  "PMU (PLL-Based, Positive-Sequence)7"/3 -> Scope13/3  "frequency"
  "PMU (PLL-Based, Positive-Sequence)7"/1 -> Scope13/1  "magnitude"
  Power Measurement (Three-Phase)7/1 -> Scope12/1
  Power Measurement (Three-Phase)6/1 -> Scope10/1
  "PMU (PLL-Based, Positive-Sequence)6"/1 -> Scope11/1  "magnitude"
  "PMU (PLL-Based, Positive-Sequence)6"/3 -> Scope11/3  "frequency"
  Power Measurement (Three-Phase)6/2 -> Scope10/2
  Bus Selector11/1 -> "PMU (PLL-Based, Positive-Sequence)6"/1, Power Measurement (Three-Phase)6/1  "<V1>"
  "PMU (PLL-Based, Positive-Sequence)6"/2 -> Scope11/2  "phase"
  Bus Selector12/1 -> Power Measurement (Three-Phase)6/2  "<I1>"
  Bus Selector10/1 -> Power Measurement (Three-Phase)5/2  "<I1>"
  "PMU (PLL-Based, Positive-Sequence)5"/2 -> Scope9/2  "phase"
  Bus Selector9/1 -> Power Measurement (Three-Phase)5/1, "PMU (PLL-Based, Positive-Sequence)5"/1  "<V1>"
  Power Measurement (Three-Phase)5/2 -> Scope8/2
  "PMU (PLL-Based, Positive-Sequence)5"/3 -> Scope9/3  "frequency"
  "PMU (PLL-Based, Positive-Sequence)5"/1 -> Scope9/1  "magnitude"
  Power Measurement (Three-Phase)5/1 -> Scope8/1
  Power Measurement (Three-Phase)11/1 -> Scope24/1
  "PMU (PLL-Based, Positive-Sequence)11"/1 -> Scope25/1  "magnitude"
  "PMU (PLL-Based, Positive-Sequence)11"/3 -> Scope25/3  "frequency"
  Power Measurement (Three-Phase)11/2 -> Scope24/2
  Bus Selector26/1 -> "PMU (PLL-Based, Positive-Sequence)11"/1, Power Measurement (Three-Phase)11/1  "<V1>"
  "PMU (PLL-Based, Positive-Sequence)11"/2 -> Scope25/2  "phase"
  Bus Selector16/1 -> Power Measurement (Three-Phase)11/2  "<I1>"
  Bus Selector18/1 -> Power Measurement (Three-Phase)12/2  "<I1>"
  "PMU (PLL-Based, Positive-Sequence)12"/2 -> Scope15/2  "phase"
  Bus Selector17/1 -> Power Measurement (Three-Phase)12/1, "PMU (PLL-Based, Positive-Sequence)12"/1  "<V1>"
  Power Measurement (Three-Phase)12/2 -> Scope14/2
  "PMU (PLL-Based, Positive-Sequence)12"/3 -> Scope15/3  "frequency"
  "PMU (PLL-Based, Positive-Sequence)12"/1 -> Scope15/1  "magnitude"
  Power Measurement (Three-Phase)12/1 -> Scope14/1
  Power Measurement (Three-Phase)13/1 -> Scope16/1
  "PMU (PLL-Based, Positive-Sequence)13"/1 -> Scope17/1  "magnitude"
  "PMU (PLL-Based, Positive-Sequence)13"/3 -> Scope17/3  "frequency"
  Power Measurement (Three-Phase)13/2 -> Scope16/2
  Bus Selector19/1 -> "PMU (PLL-Based, Positive-Sequence)13"/1, Power Measurement (Three-Phase)13/1  "<V1>"
  "PMU (PLL-Based, Positive-Sequence)13"/2 -> Scope17/2  "phase"
  Bus Selector20/1 -> Power Measurement (Three-Phase)13/2  "<I1>"
  Bus Selector25/1 -> Power Measurement (Three-Phase)10/2  "<I1>"
  "PMU (PLL-Based, Positive-Sequence)10"/2 -> Scope23/2  "phase"
  Bus Selector24/1 -> Power Measurement (Three-Phase)10/1, "PMU (PLL-Based, Positive-Sequence)10"/1  "<V1>"
  Power Measurement (Three-Phase)10/2 -> Scope22/2
  "PMU (PLL-Based, Positive-Sequence)10"/3 -> Scope23/3  "frequency"
  "PMU (PLL-Based, Positive-Sequence)10"/1 -> Scope23/1  "magnitude"
  Power Measurement (Three-Phase)10/1 -> Scope22/1
  Power Measurement (Three-Phase)9/1 -> Scope20/1
  "PMU (PLL-Based, Positive-Sequence)9"/1 -> Scope21/1  "magnitude"
  "PMU (PLL-Based, Positive-Sequence)9"/3 -> Scope21/3  "frequency"
  Power Measurement (Three-Phase)9/2 -> Scope20/2
  Bus Selector22/1 -> "PMU (PLL-Based, Positive-Sequence)9"/1, Power Measurement (Three-Phase)9/1  "<V1>"
  "PMU (PLL-Based, Positive-Sequence)9"/2 -> Scope21/2  "phase"
  Bus Selector23/1 -> Power Measurement (Three-Phase)9/2  "<I1>"
  Bus Selector21/1 -> Power Measurement (Three-Phase)8/2  "<I1>"
  "PMU (PLL-Based, Positive-Sequence)8"/2 -> Scope19/2  "phase"
  Bus Selector15/1 -> Power Measurement (Three-Phase)8/1, "PMU (PLL-Based, Positive-Sequence)8"/1  "<V1>"
  Power Measurement (Three-Phase)8/2 -> Scope18/2
  "PMU (PLL-Based, Positive-Sequence)8"/3 -> Scope19/3  "frequency"
  "PMU (PLL-Based, Positive-Sequence)8"/1 -> Scope19/1  "magnitude"
  Power Measurement (Three-Phase)8/1 -> Scope18/1
